simulink model "odd_symmetric_9"  (Simulink 6.6)
settings: Solver=ode45  StartTime=0.0  StopTime=25  RelTol=1e-3
undefined symbols (not defined in the file): A, B, D, PCIN, X, Z
libraries: xbsIndex_r4 x24
settings Model: Creator=lcrockett  LastModifiedBy=lcrockett

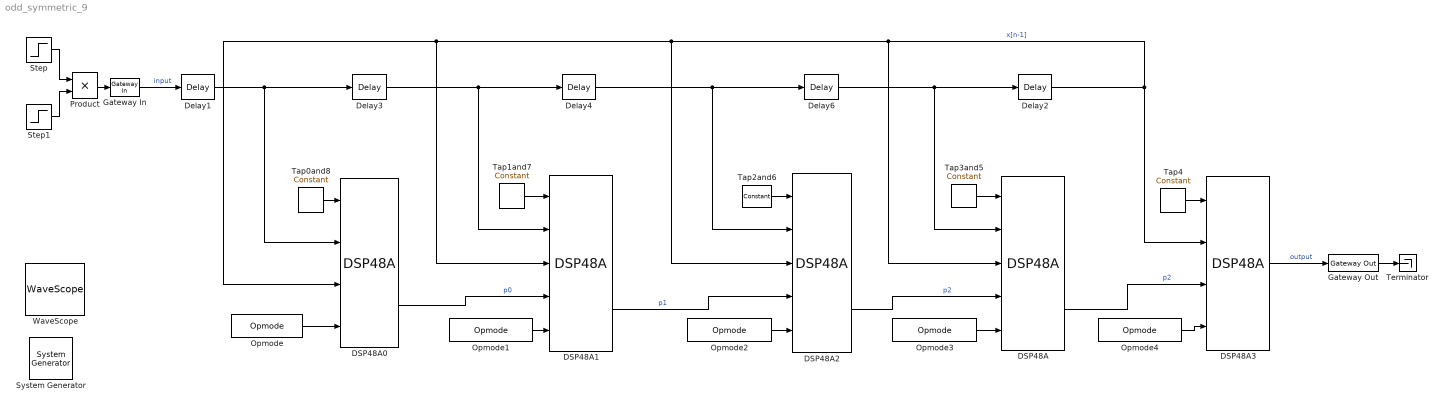
== system odd_symmetric_9 ==
  " System Generator" : xbsIndex_r4/ System Generator  Tag=genX  SystemSampleTime=-1  xilinxfamily=spartan3adsp  part=xc3sd1800a  speed=-5  package=cs484  synthesis_tool=XST  directory=./odd_symmetric_9  testbench=off  simulink_period=1  sysclk_period=10  incr_netlist=off  trim_vbits=Everywhere in SubSystem  dbl_ovrd=According to Block Masks  core_generation=According to Block Masks  run_coregen=off  deprecated_control=off  eval_field=0  block_type=sysgen
      settings: block_version=9.2.01
  DSP48A : xbsIndex_r4/DSP48A  use_op=on  use_creg=off  use_d=on  use_pcin=on  use_pcout=on  use_bcout=off  use_carryin=off  use_carryout=off  rst_all=off  en_all=off  carryin_type=Direct from carry in port  use_a0reg=on  use_a1reg=off  use_b0reg=on  use_b1reg=on  pipeline_c=on  pipeline_d=on  pipeline_mult=on  pipeline_p=on  pipeline_opmode=on  pipeline_carryin=on  rst_a=off  rst_b=off  rst_c=off  rst_d=off  rst_mult=off  rst_p=off  rst_opmode=off  rst_carry_in=off  en_a=off  en_b=off  en_c=off  en_d=off  en_mult=off  en_p=off  en_opmode=off  en_carry_in=off  dbl_ovrd=off  use_synth_model=off  device=3  block_type=dsp48a
      settings: block_version=9.2.01
  DSP48A0 : xbsIndex_r4/DSP48A  use_op=on  use_creg=off  use_d=on  use_pcin=off  use_pcout=on  use_bcout=off  use_carryin=off  use_carryout=off  rst_all=off  en_all=off  carryin_type=Direct from carry in port  use_a0reg=on  use_a1reg=off  use_b0reg=on  use_b1reg=on  pipeline_c=off  pipeline_d=on  pipeline_mult=on  pipeline_p=on  pipeline_opmode=on  pipeline_carryin=on  rst_a=off  rst_b=off  rst_c=off  rst_d=off  rst_mult=off  rst_p=off  rst_opmode=off  rst_carry_in=off  en_a=off  en_b=off  en_c=off  en_d=off  en_mult=off  en_p=off  en_opmode=off  en_carry_in=off  dbl_ovrd=off  use_synth_model=off  device=3  block_type=dsp48a
      settings: block_version=9.2.01
  DSP48A1 : xbsIndex_r4/DSP48A  use_op=on  use_creg=off  use_d=on  use_pcin=on  use_pcout=on  use_bcout=off  use_carryin=off  use_carryout=off  rst_all=off  en_all=off  carryin_type=Direct from carry in port  use_a0reg=on  use_a1reg=off  use_b0reg=on  use_b1reg=on  pipeline_c=on  pipeline_d=on  pipeline_mult=on  pipeline_p=on  pipeline_opmode=on  pipeline_carryin=on  rst_a=off  rst_b=off  rst_c=off  rst_d=off  rst_mult=off  rst_p=off  rst_opmode=off  rst_carry_in=off  en_a=off  en_b=off  en_c=off  en_d=off  en_mult=off  en_p=off  en_opmode=off  en_carry_in=off  dbl_ovrd=off  use_synth_model=off  device=3  block_type=dsp48a
      settings: block_version=9.2.01
  DSP48A2 : xbsIndex_r4/DSP48A  use_op=on  use_creg=off  use_d=on  use_pcin=on  use_pcout=on  use_bcout=off  use_carryin=off  use_carryout=off  rst_all=off  en_all=off  carryin_type=Direct from carry in port  use_a0reg=on  use_a1reg=off  use_b0reg=on  use_b1reg=on  pipeline_c=on  pipeline_d=on  pipeline_mult=on  pipeline_p=on  pipeline_opmode=on  pipeline_carryin=on  rst_a=off  rst_b=off  rst_c=off  rst_d=off  rst_mult=off  rst_p=off  rst_opmode=off  rst_carry_in=off  en_a=off  en_b=off  en_c=off  en_d=off  en_mult=off  en_p=off  en_opmode=off  en_carry_in=off  dbl_ovrd=off  use_synth_model=off  device=3  block_type=dsp48a
      settings: block_version=9.2.01
  DSP48A3 : xbsIndex_r4/DSP48A  use_op=on  use_creg=off  use_d=off  use_pcin=on  use_pcout=off  use_bcout=off  use_carryin=off  use_carryout=off  rst_all=off  en_all=off  carryin_type=Direct from carry in port  use_a0reg=on  use_a1reg=off  use_b0reg=on  use_b1reg=on  pipeline_c=on  pipeline_d=on  pipeline_mult=on  pipeline_p=on  pipeline_opmode=on  pipeline_carryin=on  rst_a=off  rst_b=off  rst_c=off  rst_d=off  rst_mult=off  rst_p=off  rst_opmode=off  rst_carry_in=off  en_a=off  en_b=off  en_c=off  en_d=off  en_mult=off  en_p=off  en_opmode=off  en_carry_in=off  dbl_ovrd=off  use_synth_model=off  device=3  block_type=dsp48a
      settings: block_version=9.2.01
  Delay{1..4,6} (5 alike) : xbsIndex_r4/Delay  en=off  latency=2  dbl_ovrd=off  reg_retiming=off  block_type=delay
      settings: block_version=9.2.01
  Gateway In : xbsIndex_r4/Gateway In  arith_type="Signed  (2's comp)"  n_bits=18  bin_pt=0  quantization="Round  (unbiased: +/- Inf)"  overflow=Saturate  period=1  dbl_ovrd=off  timing_constraint=None  locs_specified=off  LOCs={}  block_type=gatewayin
      settings: infoedit="Gateway in block.  Converts inputs of type Simulink integer, double and fixed point to  Xilinx fixed point type.<P><P>Hardware notes:  In hardware these blocks become top level input ports."  block_version=9.2.01
  Gateway Out : xbsIndex_r4/Gateway Out  hdl_port=on  timing_constraint=None  locs_specified=off  LOCs={}  block_type=gatewayout
      settings: infoedit="Gateway out block.  Converts Xilinx fixed point inputs into ouputs of type Simulink integer, double, or fixed point.<P><P>Hardware notes:  In hardware these blocks become top level output ports or are discarded, depending on how they are configured."  block_version=9.2.01
  Opmode : xbsIndex_r4/Opmode  device=DSP48A  equ=P=+(A*(D+B))  operation=Custom  logicinstr=X + Z  z_mux=0  operand=+  xy_mux=P  x_mux=A*(D+B)  carry=0  dbl_ovrd=off  block_type=opmode
      settings: block_version=9.2.01
  Opmode1 : xbsIndex_r4/Opmode  device=DSP48A  equ=P=PCIN+(A*(D+B))  operation=Custom  logicinstr=X + Z  z_mux=PCIN  operand=+  xy_mux=P  x_mux=A*(D+B)  carry=0  dbl_ovrd=off  block_type=opmode
      settings: block_version=9.2.01
  Opmode2 : xbsIndex_r4/Opmode  device=DSP48A  equ=P=PCIN+(A*(D+B))  operation=Custom  logicinstr=X + Z  z_mux=PCIN  operand=+  xy_mux=P  x_mux=A*(D+B)  carry=0  dbl_ovrd=off  block_type=opmode
      settings: block_version=9.2.01
  Opmode3 : xbsIndex_r4/Opmode  device=DSP48A  equ=P=PCIN+(A*(D+B))  operation=Custom  logicinstr=X + Z  z_mux=PCIN  operand=+  xy_mux=P  x_mux=A*(D+B)  carry=0  dbl_ovrd=off  block_type=opmode
      settings: block_version=9.2.01
  Opmode4 : xbsIndex_r4/Opmode  device=DSP48A  equ=P=PCIN+(A*B)  operation=PCIN + A*B  logicinstr=X + Z  z_mux=PCIN  operand=+  xy_mux=P  x_mux=A*(D+B)  carry=0  dbl_ovrd=off  block_type=opmode
      settings: block_version=9.2.01
  Product : Product  RndMeth=Zero
  Step : Step  Time=2  SampleTime=1
  Step1 : Step  Time=3  Before=1  After=0  SampleTime=1
  Tap0and8 : xbsIndex_r4/Constant  arith_type=Signed (2's comp)  const=16  n_bits=18  bin_pt=0  explicit_period=off  period=1  equ=P=C  opselect=C  inp2=PCIN>>17  opr=+  inp1=P  carry=CIN  dbl_ovrd=off  block_type=constant
      settings: block_version=9.2.01
  Tap1and7 : xbsIndex_r4/Constant  arith_type=Signed (2's comp)  const=-56  n_bits=18  bin_pt=0  explicit_period=off  period=1  equ=P=C  opselect=C  inp2=PCIN>>17  opr=+  inp1=P  carry=CIN  dbl_ovrd=off  block_type=constant
      settings: block_version=9.2.01
  Tap2and6 : xbsIndex_r4/Constant  arith_type=Signed (2's comp)  const=-99  n_bits=18  bin_pt=0  explicit_period=off  period=1  equ=P=C  opselect=C  inp2=PCIN>>17  opr=+  inp1=P  carry=CIN  dbl_ovrd=off  block_type=constant
      settings: block_version=9.2.01
  Tap3and5 : xbsIndex_r4/Constant  arith_type=Signed (2's comp)  const=111  n_bits=18  bin_pt=0  explicit_period=off  period=1  equ=P=C  opselect=C  inp2=PCIN>>17  opr=+  inp1=P  carry=CIN  dbl_ovrd=off  block_type=constant
      settings: block_version=9.2.01
  Tap4 : xbsIndex_r4/Constant  arith_type=Signed (2's comp)  const=10  n_bits=18  bin_pt=0  explicit_period=off  period=1  equ=P=C  opselect=C  inp2=PCIN>>17  opr=+  inp1=P  carry=CIN  dbl_ovrd=off  block_type=constant
      settings: block_version=9.2.01
  Terminator : Terminator
  WaveScope : xbsIndex_r4/WaveScope  block_type=wavescope
      settings: block_version=9.2.01
  wires:
  Opmode/1 -> DSP48A0/4
  Gateway In/1 -> Delay1/1  "input"
  Opmode1/1 -> DSP48A1/5
  Opmode2/1 -> DSP48A2/5
  Opmode3/1 -> DSP48A/5
  Delay3/1 -> DSP48A1/2, Delay4/1
  Delay4/1 -> DSP48A2/2, Delay6/1
  Delay6/1 -> DSP48A/2, Delay2/1
  DSP48A0/2 -> DSP48A1/4  "p0"
  DSP48A1/2 -> DSP48A2/4  "p1"
  DSP48A2/2 -> DSP48A/4  "p2"
  Tap2and6/1 -> DSP48A2/1
  Tap3and5/1 -> DSP48A/1
  Tap1and7/1 -> DSP48A1/1
  Tap0and8/1 -> DSP48A0/1
  Gateway Out/1 -> Terminator/1
  Product/1 -> Gateway In/1
  Step/1 -> Product/1
  Step1/1 -> Product/2
  Delay1/1 -> DSP48A0/2, Delay3/1
  Opmode4/1 -> DSP48A3/4
  Tap4/1 -> DSP48A3/1
  DSP48A/2 -> DSP48A3/3  "p2"
  DSP48A3/1 -> Gateway Out/1  "output"
  Delay2/1 -> DSP48A3/2, DSP48A/3, DSP48A2/3, DSP48A1/3, DSP48A0/3  "x[n-1]"
